simulink model "controller"  (R2018a)
settings: Solver=VariableStepAuto  StartTime=0.0  StopTime=30  RelTol=1e-3  EnableMultiTasking=on
values from neighbouring files (symbols this model uses):
  g = 9.81    [controller_script.m]
  I = [0.06 0.003 0.0006;0.003 0.05 0.002;0.002 0.003 0.1]    [controller_script.m]
  Kp = 15*eye(3)    [controller_script.m]
  Kr = 20*eye(3)    [controller_script.m]
  Kv = 10*eye(3)    [controller_script.m]
  Kw = 2*eye(3)    [controller_script.m]
  m = 1.5    [controller_script.m]
  zw = [0;0;1]    [controller_script.m]
libraries: simulink x3
settings Model: Creator=hugoa  LastModifiedBy=ALEX
settings OptimizationCC: LifeSpan=inf
settings DebuggingCC: SFUnexpectedBacktrackingDiag=warning  SFNoUnconditionalDefaultTransitionDiag=warning  SFExecutionAtInitializationDiag=none
settings CodeAppCC: StateflowObjectComments=on
settings GRTTargetCC: TargetLangStandard=C89/C90 (ANSI)  GeneratePreprocessorConditionals=Disable all
settings ConfigComp: CovMetricSettings=dw  CovHtmlReporting=on  CovSaveCumulativeToWorkspaceVar=on  CovSaveSingleToWorkspaceVar=on  CovExternalEMLEnable=off

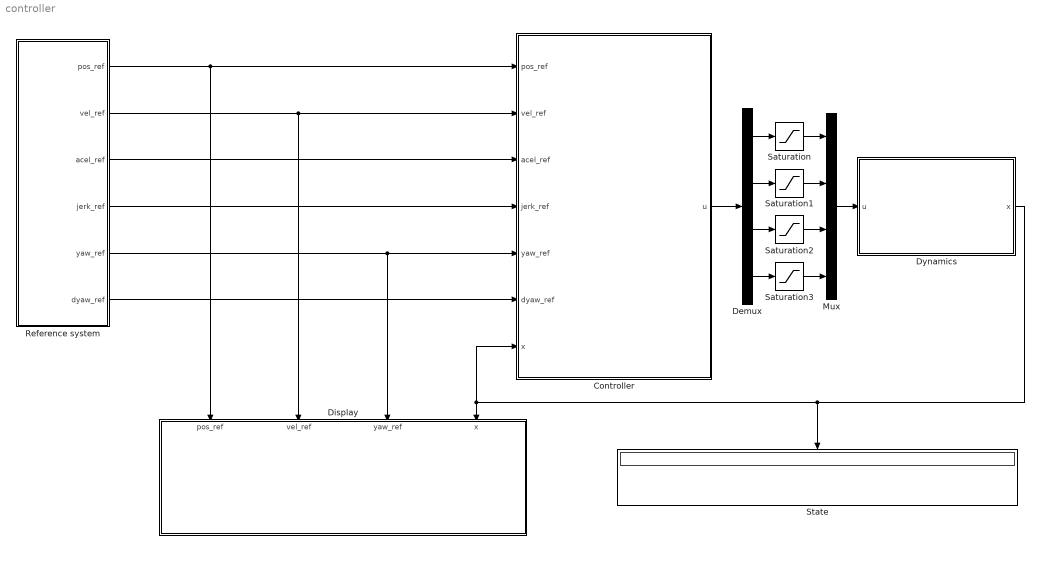
== system controller ==
  "Controller " : Subsystem
  Demux : Demux
  Display : Subsystem
  Dynamics : Subsystem
  Mux : Mux
  Reference system : Subsystem
  Saturation : Saturate  UpperLimit=1000  LowerLimit=-100
  Saturation1 : Saturate  UpperLimit=1000  LowerLimit=-100
  Saturation2 : Saturate  UpperLimit=100  LowerLimit=-100
  Saturation3 : Saturate  UpperLimit=100  LowerLimit=-100
  State : Display
  wires:
  Dynamics/1(x) -> State/1, "Controller "/7(x), Display/4(x)
  Reference system/1(pos_ref) -> Display/1(pos_ref), "Controller "/1(pos_ref)
  Reference system/2(vel_ref) -> Display/2(vel_ref), "Controller "/2(vel_ref)
  Reference system/3(acel_ref) -> "Controller "/3(acel_ref)
  Reference system/4(jerk_ref) -> "Controller "/4(jerk_ref)
  Reference system/5(yaw_ref) -> Display/3(yaw_ref), "Controller "/5(yaw_ref)
  Reference system/6(dyaw_ref) -> "Controller "/6(dyaw_ref)
  "Controller "/1(u) -> Demux/1
  Demux/1 -> Saturation/1
  Demux/2 -> Saturation1/1
  Demux/3 -> Saturation2/1
  Demux/4 -> Saturation3/1
  Saturation3/1 -> Mux/4
  Saturation/1 -> Mux/1
  Saturation1/1 -> Mux/2
  Saturation2/1 -> Mux/3
  Mux/1 -> Dynamics/1(u)

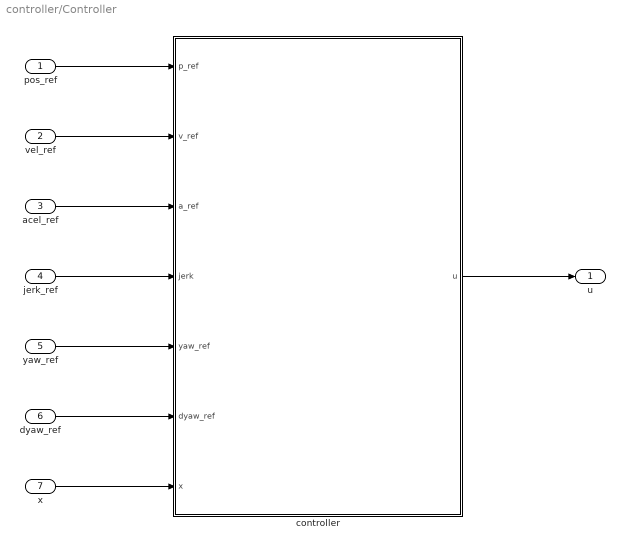
== system controller/Controller  ==
  pos_ref : Inport
  vel_ref : Inport  Port=2
  acel_ref : Inport  Port=3
  jerk_ref : Inport  Port=4
  yaw_ref : Inport  Port=5
  dyaw_ref : Inport  Port=6
  x : Inport  Port=7
  controller : MATLAB Function  TreatAsAtomicUnit=on
  u : Outport
  wires:
  pos_ref/1 -> controller/1(p_ref)
  controller/1(u) -> u/1
  x/1 -> controller/7(x)
  vel_ref/1 -> controller/2(v_ref)
  acel_ref/1 -> controller/3(a_ref)
  jerk_ref/1 -> controller/4(jerk)
  yaw_ref/1 -> controller/5(yaw_ref)
  dyaw_ref/1 -> controller/6(dyaw_ref)

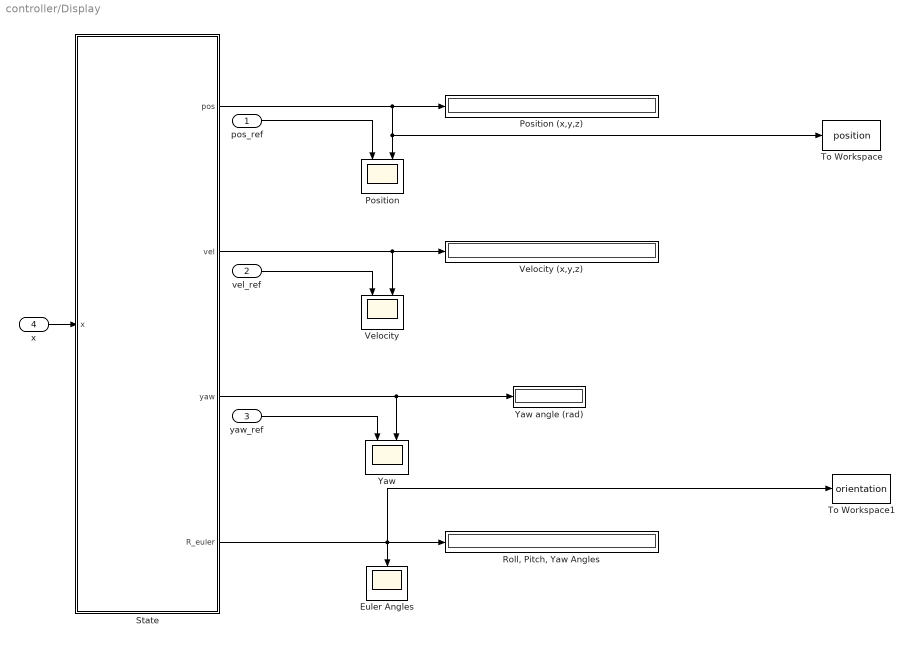
== system controller/Display ==
  pos_ref : Inport
  vel_ref : Inport  Port=2
  yaw_ref : Inport  Port=3
  x : Inport  Port=4
  Euler Angles : Scope
  Position : Scope  NumInputPorts=2
  Position (x,y,z) : Display
  "Roll, Pitch, Yaw Angles" : Display
  State : MATLAB Function  TreatAsAtomicUnit=on
  To Workspace : ToWorkspace  VariableName=position  SaveFormat=Timeseries  SampleTime=-1
  To Workspace1 : ToWorkspace  VariableName=orientation  SaveFormat=Timeseries  SampleTime=-1
  Velocity : Scope  NumInputPorts=2
  Velocity (x,y,z) : Display
  Yaw : Scope  NumInputPorts=2
  Yaw angle (rad) : Display
  wires:
  yaw_ref/1 -> Yaw/1
  x/1 -> State/1(x)
  State/3(yaw) -> Yaw/2, Yaw angle (rad)/1
  State/4(R_euler) -> To Workspace1/1, "Roll, Pitch, Yaw Angles"/1, Euler Angles/1
  vel_ref/1 -> Velocity/1
  State/2(vel) -> Velocity (x,y,z)/1, Velocity/2
  State/1(pos) -> To Workspace/1, Position/2, Position (x,y,z)/1
  pos_ref/1 -> Position/1

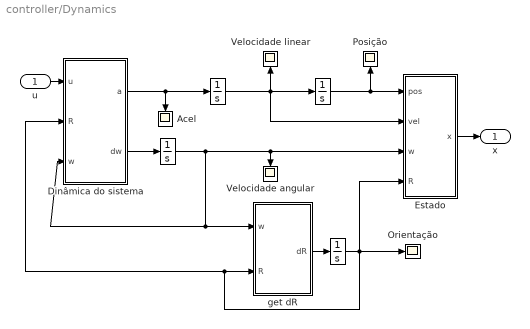
== system controller/Dynamics ==
  u : Inport
  " " : Integrator  InitialCondition=[0;0;0]
  " " : Integrator  InitialCondition=[0;0;0]
  " " : Integrator  InitialCondition=eye(3)  UpperSaturationLimit=1  LowerSaturationLimit=0
  " " : Integrator  InitialCondition=[0;0;0]
  Acel : Scope
  Dinâmica do sistema : MATLAB Function  TreatAsAtomicUnit=on
  Estado : MATLAB Function  TreatAsAtomicUnit=on
  Orientação : Scope
  Posição : Scope
  Velocidade angular : Scope
  Velocidade linear : Scope
  get dR : MATLAB Function  TreatAsAtomicUnit=on
  x : Outport
  wires:
  Dinâmica do sistema/2(dw) -> " "/1
  Dinâmica do sistema/1(a) -> Acel/1, " "/1
  " "/1 -> Velocidade angular/1, Estado/3(w), Dinâmica do sistema/3(w), get dR/1(w)
  " "/1 -> Estado/2(vel), " "/1, Velocidade linear/1
  " "/1 -> Estado/1(pos), Posição/1
  Estado/1(x) -> x/1
  get dR/1(dR) -> " "/1
  u/1 -> Dinâmica do sistema/1(u)
  " "/1 -> get dR/2(R), Dinâmica do sistema/2(R), Orientação/1, Estado/4(R)

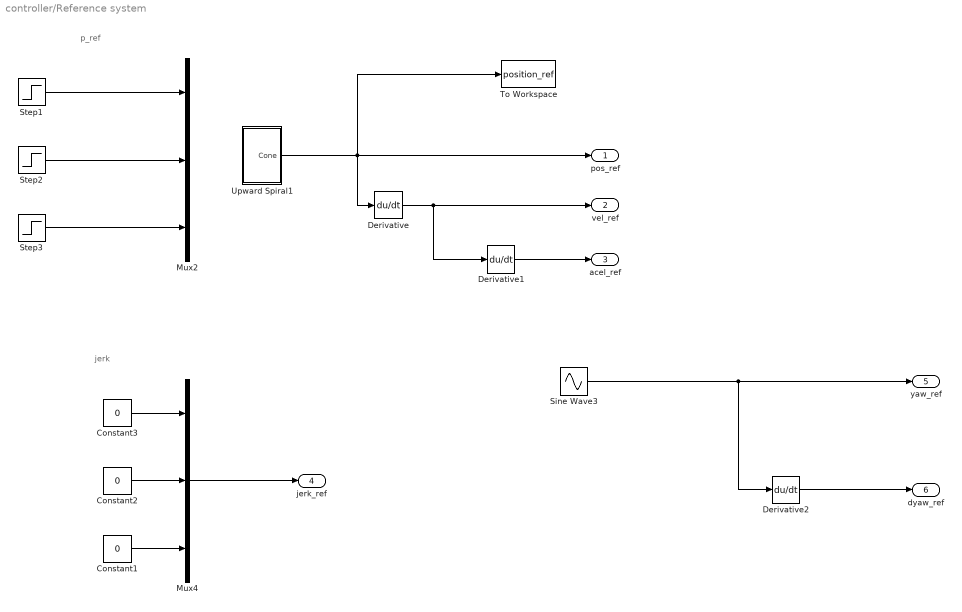
== system controller/Reference system ==
  note: jerk
  note: p_ref
  Constant1 : Constant  Value=0
  Constant2 : Constant  Value=0
  Constant3 : Constant  Value=0
  Derivative : Derivative  CoefficientInTFapproximation=0.01
  Derivative1 : Derivative  CoefficientInTFapproximation=0.01
  Derivative2 : Derivative  CoefficientInTFapproximation=0.01
  Mux2 : Mux  Inputs=3
  Mux4 : Mux  Inputs=3
  Sine Wave3 : Sin  SampleTime=0
  Step1 : Step  After=2  SampleTime=0
  Step2 : Step  After=3  SampleTime=0
  Step3 : Step  SampleTime=0
  To Workspace : ToWorkspace  VariableName=position_ref  SaveFormat=Timeseries  SampleTime=-1
  Upward Spiral1 : Subsystem
  pos_ref : Outport
  vel_ref : Outport  Port=2
  acel_ref : Outport  Port=3
  jerk_ref : Outport  Port=4
  yaw_ref : Outport  Port=5
  dyaw_ref : Outport  Port=6
  wires:
  Sine Wave3/1 -> Derivative2/1, yaw_ref/1
  Constant3/1 -> Mux4/1
  Constant1/1 -> Mux4/3
  Constant2/1 -> Mux4/2
  Derivative/1 -> vel_ref/1, Derivative1/1
  Derivative1/1 -> acel_ref/1
  Derivative2/1 -> dyaw_ref/1
  Mux4/1 -> jerk_ref/1
  Step1/1 -> Mux2/1
  Step2/1 -> Mux2/2
  Step3/1 -> Mux2/3
  Upward Spiral1/1(Cone) -> Derivative/1, To Workspace/1, pos_ref/1

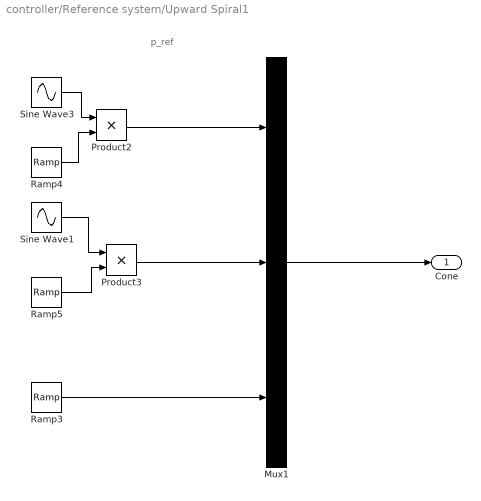
== system controller/Reference system/Upward Spiral1 ==
  note: p_ref
  Mux1 : Mux  Inputs=3
  Product2 : Product
  Product3 : Product
  Ramp3 : simulink/Sources/Ramp  slope=0.5  start=1  InitialOutput=0
  Ramp4 : simulink/Sources/Ramp  slope=0.5  start=1  InitialOutput=0
  Ramp5 : simulink/Sources/Ramp  slope=0.5  start=1  InitialOutput=1
  Sine Wave1 : Sin  Frequency=2  Phase=pi/2  SampleTime=0
  Sine Wave3 : Sin  Frequency=2  SampleTime=0
  Cone : Outport
  wires:
  Sine Wave1/1 -> Product3/1
  Product3/1 -> Mux1/2
  Ramp3/1 -> Mux1/3
  Ramp5/1 -> Product3/2
  Ramp4/1 -> Product2/2
  Product2/1 -> Mux1/1
  Mux1/1 -> Cone/1
  Sine Wave3/1 -> Product2/1

== matlab function controller/Dynamics/get dR ==
  data: dR output; w input; R input
function dR = fcn(w, R)
%#codegen
skew_w = [0,-w(3),w(2); w(3),0,-w(1); -w(2),w(1),0];



dR = R*skew_w;

== matlab function controller/Dynamics/Dinâmica do sistema ==
  data: u input; R input; a output; w input size=3; dw output; I parameter; g parameter; m parameter
function [a,dw] = fcn(u,R,w, I, g, m)
%#codegen
zw = [0;0;1];
zB = R*zw;

skew_w = [0,-w(3),w(2); w(3),0,-w(1); -w(2),w(1),0];
uT = [u(2);u(3);u(4)];



a = -g*zw+(u(1)/m)*zB;
%dw = inv(I)*(-skew_w*I*w + uT);
dw = I\((cross(-w,I*w))+uT);

== matlab function controller/Dynamics/Estado ==
  data: pos input; vel input; w input; R input; x output
function x = fcn(pos, vel, w, R)
%#codegen

x = [pos, vel, w, R];

== matlab function controller/Controller /controller ==
  data: p_ref input; v_ref input; a_ref input; jerk input; yaw_ref input; dyaw_ref input; u output; x input; Kp parameter; g parameter; Kr parameter; m parameter; zw parameter; Kv parameter; Kw parameter
function u    = fcn(p_ref, v_ref, a_ref, jerk, yaw_ref, dyaw_ref, x, Kp, g, Kr, m, zw, Kv, Kw)

%% GET THE STATE
    %Position
    p = x(1:3,1);
    %Velocity
    v = x(1:3,2);
    %Angular velocity
    wb = x(1:3,3);
    %Rotation matrix
    R = x(1:3,4:6);
    %R_euler = rotm2eul(R);

%%%%%%%%%%%%%%%%%%%%%%%%%%%%%%%%%%%%%%%%%%%%%%%

%% ERRORS

    %Position Error
    ep = p - p_ref;
    %Velocity Error
    ev = v - v_ref;

%%%%%%%%%%%%%%%%%%%%%%%%%%%%%%%%%%%%%%%%%%%%%%%

%% EQUATIONS

    F_des = -Kp*ep - Kv*ev + m*g*zw + m*a_ref;

    zB = R*zw;
    u1= dot(F_des, zB);

    %Rotation matrix
    zB_des = F_des/norm(F_des);
    xA_des = [cos(yaw_ref); sin(yaw_ref); 0];
    yB_des = cross(zB_des,xA_des)/norm(cross(zB_des,xA_des));
    xB_des = cross(yB_des,zB_des);
    R_des = [xB_des, yB_des, zB_des];
    
    %Orientation Error
    eR_aux = (transpose(R_des)*R - transpose(R)*R_des);
    eR = 0.5 * [eR_aux(3,2); eR_aux(1,3); eR_aux(2,1)];

    %Angular velocity
    h = m/u1*(jerk - ( dot(zB_des, jerk)*zB_des));
    p_des = dot(-h,yB_des);
    q_des = dot(h,xB_des);
    % VERY BAD
    w_aux = R\[xA_des yB_des zw]*[0;0;dyaw_ref];
    r_des = w_aux(3);

    wb_ref = [p_des; q_des; r_des];
    
    %Angular Velocity Error
    ew = wb - wb_ref; 

    
%%%%%%%%%%%%%%%%%%%%%%%%%%%%%%%%%%%%%%%%%%%%%%%

%% Limit yaw angle to pi/6 = 30º
    R_des_euler = rotm2eul(R_des);
    if(R_des_euler(3)>pi/6)
        R_des_euler(3) = pi/6;
    end
    if(R_des_euler(3)<-pi/6)
        R_des_euler(3) = -pi/6;
    end

%% OUTPUT

    uT = - Kr*eR - Kw*ew;
    u = [u1; uT];
%%%%%%%%%%%%%%%%%%%%%%%%%%%%%%%%%%%%%%%%%%%%%%%

== matlab function controller/Display/State ==
  data: x input; pos output; vel output; yaw output; R_euler output
function [pos, vel, yaw, R_euler] = fcn(x)
%#codegen


 R = x(1:3,4:6);
 R_euler_aux = rotm2eul(R);
 %R_euler(1)    ->  Z   ->  Yaw
 %R_euler(2)    ->  X   ->  Roll
 %R_euler(3)    ->  Y   ->  Pitch
 R_euler = [R_euler_aux(2); R_euler_aux(3); R_euler_aux(1)];
 
 
% OUTPUT
pos = x(1:3,1);
vel = x(1:3,2);
yaw = R_euler(3);
